simulink model "buck_02_bis_2018_b"  (R2018b)
settings: Solver=ode45  StartTime=0.0  StopTime=400/F  MaxStep=1/(10*F)  RelTol=1e-3  EnableMultiTasking=on
values from neighbouring files (symbols this model uses):
  C = 9.3e-6    (= 9.3e-06)    [buck_01_script.m]    (also in buck_02_script.m; buck_04_script.m)
  C1 = 5.5e-6    (= 5.5e-06)    [buck_01_script.m]    (also in buck_02_script.m; buck_04_script.m)
  duty = Vs / Ve    (= 0.66)    [buck_01_script.m]    (also in buck_02_script.m; buck_04_script.m)
  F = 500e3    (= 500000)    [buck_01_script.m]    (also in buck_02_script.m; buck_04_script.m)
  L = 1.9e-6    (= 1.9e-06)    [buck_01_script.m]    (also in buck_02_script.m; buck_04_script.m)
  L1 = 5e-6    (= 5e-06)    [buck_01_script.m]    (also in buck_02_script.m; buck_04_script.m)
  R = Vs^2 / Ps    (= 5.445)    [buck_01_script.m]    (also in buck_02_script.m = 0.5445; buck_04_script.m)
  Ve = 5    [buck_01_script.m]    (also in buck_02_script.m; buck_04_script.m)
libraries: powerlib x31
settings Model: Creator=lefrancp  LastModifiedBy=lefrancp
settings DataIOCC: LimitDataPoints=on  SaveFormat=Array
settings OptimizationCC: LifeSpan=inf
settings DebuggingCC: SolverPrmCheckMsg=warning  SFUnexpectedBacktrackingDiag=warning  SFNoUnconditionalDefaultTransitionDiag=warning  SFExecutionAtInitializationDiag=none
settings HardwareCC: ProdBitPerPointer=32  ProdBitPerSizeT=32  ProdBitPerPtrDiffT=32  ProdLargestAtomicFloat=None  ProdIntDivRoundTo=Undefined  ProdEndianess=Unspecified  ProdWordSize=32  ProdHWDeviceType=32-bit Generic
settings ModelReferenceCC: PropagateSignalLabelsOutOfModel=off
settings SFSimCC: SimUseLocalCustomCode=off
settings RTWCC: RTWUseLocalCustomCode=off
settings CodeAppCC: StateflowObjectComments=on
settings GRTTargetCC: TargetLangStandard=C89/C90 (ANSI)  GeneratePreprocessorConditionals=Disable all
settings ConfigComp: CovMetricSettings=dw  CovHtmlReporting=on  CovSaveCumulativeToWorkspaceVar=on  CovSaveSingleToWorkspaceVar=on  CovExternalEMLEnable=off  CovSFcnEnable=off
settings SimscapeCC: SimscapeNormalizeSystem=off

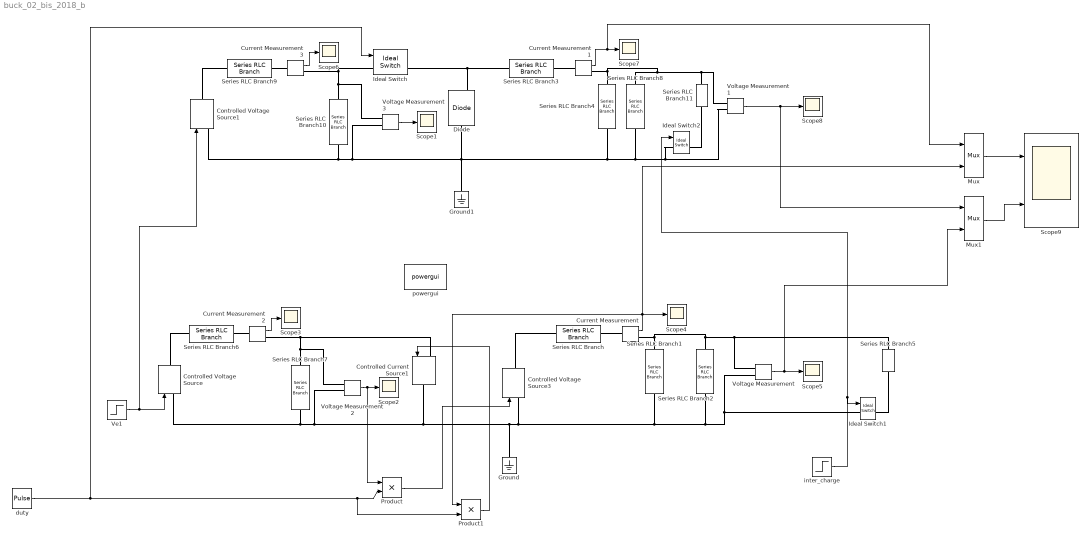
== system buck_02_bis_2018_b ==
  Controlled Current Source1 : powerlib/Electrical Sources/Controlled Current Source  Initialize=on  Source_Type=AC  Amplitude=0  Phase=0  Frequency=0  Measurements=None
      settings: SourceProductName=Simscape Electrical
  Controlled Voltage Source : powerlib/Electrical Sources/Controlled Voltage Source  Initialize=on  Source_Type=AC  Amplitude=0  Phase=0  Frequency=0  Measurements=None
      settings: SourceProductName=Simscape Electrical
  Controlled Voltage Source1 : powerlib/Electrical Sources/Controlled Voltage Source  Initialize=on  Source_Type=AC  Amplitude=0  Phase=0  Frequency=0  Measurements=None
      settings: SourceProductName=Simscape Electrical
  Controlled Voltage Source3 : powerlib/Electrical Sources/Controlled Voltage Source  Initialize=on  Source_Type=AC  Amplitude=0  Phase=0  Frequency=0  Measurements=None
      settings: SourceProductName=Simscape Electrical
  Current Measurement{,1..3} (4 alike) : powerlib/Measurements/Current Measurement  PhasorSimulation=off  OutputType=Complex  PSBequivalent=0
      settings: SourceProductName=Simscape Electrical
  Diode : powerlib/Power Electronics/Diode  Ron=0.001  Lon=0  Vf=0.01  IC=0  UseSnubber=off  Rs=500  Cs=250e-9  Measurements=on
      settings: SourceProductName=Simscape Electrical
  Ground : powerlib/Elements/Ground  LConnTagsString=a
      settings: SourceProductName=Simscape Electrical
  Ground1 : powerlib/Elements/Ground  LConnTagsString=a
      settings: SourceProductName=Simscape Electrical
  Ideal Switch : powerlib/Power Electronics/Ideal Switch  Ron=0.001  Lon=0  IC=0  Rs=1e5  Cs=inf  Measurements=on
      settings: SourceProductName=Simscape Electrical
  Ideal Switch1 : powerlib/Power Electronics/Ideal Switch  Ron=0.001  Lon=0  IC=0  Rs=1e5  Cs=inf  Measurements=on
      settings: SourceProductName=Simscape Electrical
  Ideal Switch2 : powerlib/Power Electronics/Ideal Switch  Ron=0.001  Lon=0  IC=0  Rs=1e5  Cs=inf  Measurements=on
      settings: SourceProductName=Simscape Electrical
  Mux : Mux  Inputs=2
  Mux1 : Mux  Inputs=2
  Product : Product
  Product1 : Product
  Scope{1..8} (8 alike) : Scope
  Scope9 : Scope  NumInputPorts=2
  Series RLC Branch : powerlib/Elements/Series RLC Branch  LConnTagsString=__new0  RConnTagsString=__new0  BranchType=L  Resistance=1  Inductance=L  SetiL0=off  InitialCurrent=0  Capacitance=1e-6  Setx0=off  InitialVoltage=0  Measurements=None
      settings: SourceProductName=Simscape Electrical
  Series RLC Branch1 : powerlib/Elements/Series RLC Branch  LConnTagsString=__new0  RConnTagsString=__new0  BranchType=C  Resistance=1  Inductance=L  SetiL0=off  InitialCurrent=0  Capacitance=C  Setx0=off  InitialVoltage=0  Measurements=None
      settings: SourceProductName=Simscape Electrical
  Series RLC Branch10 : powerlib/Elements/Series RLC Branch  LConnTagsString=__new0  RConnTagsString=__new0  BranchType=C  Resistance=1  Inductance=L  SetiL0=off  InitialCurrent=0  Capacitance=C1  Setx0=off  InitialVoltage=0  Measurements=None
      settings: SourceProductName=Simscape Electrical
  Series RLC Branch11 : powerlib/Elements/Series RLC Branch  LConnTagsString=__new0  RConnTagsString=__new0  BranchType=R  Resistance=R*3  Inductance=L  SetiL0=off  InitialCurrent=0  Capacitance=C  Setx0=off  InitialVoltage=0  Measurements=None
      settings: SourceProductName=Simscape Electrical
  Series RLC Branch2 : powerlib/Elements/Series RLC Branch  LConnTagsString=__new0  RConnTagsString=__new0  BranchType=R  Resistance=R  Inductance=L  SetiL0=off  InitialCurrent=0  Capacitance=C  Setx0=off  InitialVoltage=0  Measurements=None
      settings: SourceProductName=Simscape Electrical
  Series RLC Branch3 : powerlib/Elements/Series RLC Branch  LConnTagsString=__new0  RConnTagsString=__new0  BranchType=L  Resistance=1  Inductance=L  SetiL0=off  InitialCurrent=0  Capacitance=1e-6  Setx0=off  InitialVoltage=0  Measurements=None
      settings: SourceProductName=Simscape Electrical
  Series RLC Branch4 : powerlib/Elements/Series RLC Branch  LConnTagsString=__new0  RConnTagsString=__new0  BranchType=C  Resistance=1  Inductance=L  SetiL0=off  InitialCurrent=0  Capacitance=C  Setx0=off  InitialVoltage=0  Measurements=None
      settings: SourceProductName=Simscape Electrical
  Series RLC Branch5 : powerlib/Elements/Series RLC Branch  LConnTagsString=__new0  RConnTagsString=__new0  BranchType=R  Resistance=R*3  Inductance=L  SetiL0=off  InitialCurrent=0  Capacitance=C  Setx0=off  InitialVoltage=0  Measurements=None
      settings: SourceProductName=Simscape Electrical
  Series RLC Branch6 : powerlib/Elements/Series RLC Branch  LConnTagsString=__new0  RConnTagsString=__new0  BranchType=L  Resistance=1  Inductance=L1  SetiL0=off  InitialCurrent=0  Capacitance=1e-6  Setx0=off  InitialVoltage=0  Measurements=None
      settings: SourceProductName=Simscape Electrical
  Series RLC Branch7 : powerlib/Elements/Series RLC Branch  LConnTagsString=__new0  RConnTagsString=__new0  BranchType=C  Resistance=1  Inductance=L  SetiL0=off  InitialCurrent=0  Capacitance=C1  Setx0=off  InitialVoltage=0  Measurements=None
      settings: SourceProductName=Simscape Electrical
  Series RLC Branch8 : powerlib/Elements/Series RLC Branch  LConnTagsString=__new0  RConnTagsString=__new0  BranchType=R  Resistance=R  Inductance=L  SetiL0=off  InitialCurrent=0  Capacitance=C  Setx0=off  InitialVoltage=0  Measurements=None
      settings: SourceProductName=Simscape Electrical
  Series RLC Branch9 : powerlib/Elements/Series RLC Branch  LConnTagsString=__new0  RConnTagsString=__new0  BranchType=L  Resistance=1  Inductance=L1  SetiL0=off  InitialCurrent=0  Capacitance=1e-6  Setx0=off  InitialVoltage=0  Measurements=None
      settings: SourceProductName=Simscape Electrical
  Ve1 : Step  Time=1e-4  Before=Ve  After=Ve+0.1  SampleTime=0
  Voltage Measurement{,1..3} (4 alike) : powerlib/Measurements/Voltage Measurement  PhasorSimulation=off  OutputType=Complex  PSBequivalent=0
      settings: SourceProductName=Simscape Electrical
  duty : DiscretePulseGenerator  PulseType=Time based  Period=1/F  PulseWidth=duty*100
  inter_charge : Step  Time=2e-4  SampleTime=0
  powergui : powerlib/powergui  Priority=1  SimulationMode=Continuous  SampleTime=50e-6  frequency=60  Iterations=50  frequencyindice=0  Pbase=100e6  ErrMax=1e-4  UnitsV=kV  UnitsW=MW  buscounter=0  FunctionMessages=off  echomessages=off  EnableUseOfTLC=off  CurrentSourceSwitches=on  DisableSnubberDevices=off  DisableRonSwitches=off  DisableVfSwitches=off  DisplayEquations=off  AutomaticDiscreteSolvers=off  SolverType=Tustin  Interpol=off  ExternalGateDelay=off  methode=off  Ts=0  x0status=blocks  SPID=off  SwTol=0  HookPort=off  NonlinearTolerance=0  nMaxIteration=15  ContinueOnMaxIteration=off  RestoreLinks=warning  ResistiveCurrentMeasurement=off  Frange=[0:2:500]  Ylog=off  Xlog=on  ShowGrid=off  save=off  variable=ZData  structure=0  ZoomFFT=off  StartTime=0.0  cycles=1  DisplayStyle=1  fundamental=60  FreqAxis=off  MaxFrequency=1000  frequencyindicesteady=1  RmsSteady=1  display=off
      settings: SourceProductName=Simscape Electrical
  wires:
  Voltage Measurement/1 -> Mux1/2, Scope5/1
  Current Measurement/1 -> Mux/2, Product1/1, Scope4/1
  Voltage Measurement2/1 -> Product/1, Scope2/1
  Current Measurement2/1 -> Scope3/1
  Product/1 -> Controlled Voltage Source3/1
  Product1/1 -> Controlled Current Source1/1
  Current Measurement1/1 -> Mux/1, Scope7/1
  Ve1/1 -> Controlled Voltage Source1/1, Controlled Voltage Source/1
  Voltage Measurement1/1 -> Mux1/1, Scope8/1
  duty/1 -> Ideal Switch/1, Product1/2, Product/2
  Current Measurement3/1 -> Scope6/1
  Voltage Measurement3/1 -> Scope1/1
  inter_charge/1 -> Ideal Switch2/1, Ideal Switch1/1
  Mux1/1 -> Scope9/2
  Mux/1 -> Scope9/1
  connections:
  Ground/LConn1 -- Controlled Voltage Source3/LConn1 -- Series RLC Branch1/RConn1 -- Ideal Switch1/LConn1 -- Voltage Measurement/LConn2 -- Series RLC Branch2/RConn1 -- Controlled Current Source1/RConn1 -- Voltage Measurement2/LConn2 -- Series RLC Branch7/RConn1 -- Controlled Voltage Source/LConn1
  Controlled Voltage Source3/RConn1 -- Series RLC Branch/LConn1
  Series RLC Branch1/LConn1 -- Current Measurement/RConn1 -- Series RLC Branch5/LConn1 -- Voltage Measurement/LConn1 -- Series RLC Branch2/LConn1
  Series RLC Branch7/LConn1 -- Voltage Measurement2/LConn1 -- Controlled Current Source1/LConn1 -- Current Measurement2/RConn1
  Series RLC Branch/RConn1 -- Current Measurement/LConn1
  Series RLC Branch6/LConn1 -- Controlled Voltage Source/RConn1
  Current Measurement2/LConn1 -- Series RLC Branch6/RConn1
  Ideal Switch1/RConn1 -- Series RLC Branch5/RConn1
  Series RLC Branch10/LConn1 -- Voltage Measurement3/LConn1 -- Ideal Switch/LConn1 -- Current Measurement3/RConn1
  Series RLC Branch11/LConn1 -- Series RLC Branch8/LConn1 -- Current Measurement1/RConn1 -- Series RLC Branch4/LConn1 -- Voltage Measurement1/LConn1
  Series RLC Branch8/RConn1 -- Series RLC Branch4/RConn1 -- Voltage Measurement3/LConn2 -- Series RLC Branch10/RConn1 -- Controlled Voltage Source1/LConn1 -- Ground1/LConn1 -- Diode/LConn1 -- Ideal Switch2/LConn1 -- Voltage Measurement1/LConn2
  Series RLC Branch3/LConn1 -- Ideal Switch/RConn1 -- Diode/RConn1
  Series RLC Branch9/LConn1 -- Controlled Voltage Source1/RConn1
  Ideal Switch2/RConn1 -- Series RLC Branch11/RConn1
  Current Measurement3/LConn1 -- Series RLC Branch9/RConn1
  Series RLC Branch3/RConn1 -- Current Measurement1/LConn1
